simulink model "CruiseControl"  (R2020a)
settings: Solver=VariableStepAuto  StartTime=0.0  StopTime=120  RelTol=1e-3
values from neighbouring files (symbols this model uses):
  b = 50.0    [cruisectrl.sldd]
  Ki = 40.0    [cruisectrl.sldd]
  Kp = 800.0    [cruisectrl.sldd]
  M = 1000.0    [cruisectrl.sldd]
settings Model: DataDictionary=cruisectrl.sldd  Creator=USER  LastModifiedBy=USER

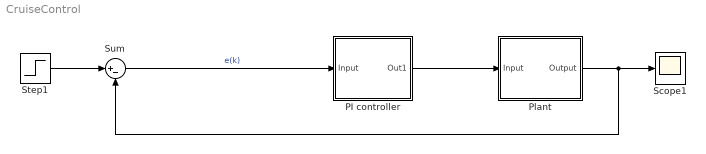
== system CruiseControl ==
  PI controller : Subsystem
  Plant : Subsystem
  Scope1 : Scope
  Step1 : Step  After=500  SampleTime=0
  Sum : Sum  Inputs=|+-
  wires:
  Sum/1 -> PI controller/1(Input)  "e(k)"
  Step1/1 -> Sum/1
  Plant/1(Output) -> Scope1/1, Sum/2
  PI controller/1(Out1) -> Plant/1(Input)

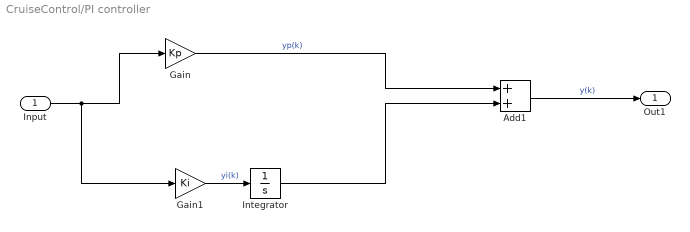
== system CruiseControl/PI controller ==
  Input : Inport
  Add1 : Sum
  Gain : Gain  Gain=Kp
  Gain1 : Gain  Gain=Ki
  Integrator : Integrator
  Out1 : Outport
  wires:
  Add1/1 -> Out1/1  "y(k)"
  Gain/1 -> Add1/1  "yp(k)"
  Input/1 -> Gain1/1, Gain/1
  Gain1/1 -> Integrator/1  "yi(k)"
  Integrator/1 -> Add1/2

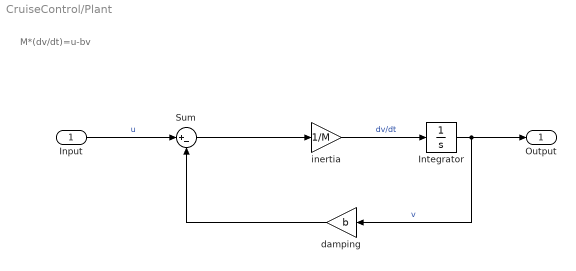
== system CruiseControl/Plant ==
  note: M*(dv/dt)=u-bv
  Input : Inport
  Integrator : Integrator
  Sum : Sum  Inputs=|+-
  damping : Gain  Gain=b
  inertia : Gain  Gain=1/M
  Output : Outport
  wires:
  damping/1 -> Sum/2
  inertia/1 -> Integrator/1  "dv/dt"
  Input/1 -> Sum/1  "u"
  Integrator/1 -> Output/1, damping/1  "v"
  Sum/1 -> inertia/1
